simulink model "IEEE_39_bus_steady_state"  (R2021b)
settings: Solver=ode3  StartTime=0.0  StopTime=10  FixedStep=Ts  MaxStep=1/60  RelTol=1e-2  AbsTol=1e-1
PreLoadFcn:
  | Ts=50e-6; ssn_ieee39_params; dec=20;
InitFcn:
  | Ts=50e-6; ssn_ieee39_params; dec=20;
values from neighbouring files (symbols this model uses):
  f = 50    [ssn_ieee39_params_ctrl.m]
  fNom = f    (= 60)    [ssn_ieee39_params_ctrl.m]
  ILR = 5.02    [ssn_ieee39_params_ctrl.m]
  IQMIN = 0.1    [ssn_ieee39_params_ctrl.m]
  ISCLIM = 1    [ssn_ieee39_params_ctrl.m]
  ITFpu = 1.10    (= 1.1)    [ssn_ieee39_params_ctrl.m]
  K = 1    [ssn_ieee39_params_ctrl.m]
  K1 = 1    [ssn_ieee39_params_ctrl.m]
  K2 = 2    [ssn_ieee39_params_ctrl.m]
  KCL = 1.04    [ssn_ieee39_params_ctrl.m]
  KFB = 0    [ssn_ieee39_params_ctrl.m]
  KFF = 1    [ssn_ieee39_params_ctrl.m]
  KFIX = 1    [ssn_ieee39_params_ctrl.m]
  KG = 1    [ssn_ieee39_params_ctrl.m]
  KIA = 59.91    [ssn_ieee39_params_ctrl.m]
  KIOEX = 0.0303    [ssn_ieee39_params_ctrl.m]
  KIUEX = 0.0303    [ssn_ieee39_params_ctrl.m]
  KIUOEX = 1    [ssn_ieee39_params_ctrl.m]
  KIUUEX = 1    [ssn_ieee39_params_ctrl.m]
  KLR = 22.47    [ssn_ieee39_params_ctrl.m]
  KM = 1    [ssn_ieee39_params_ctrl.m]
  KOEL = 0.24    [ssn_ieee39_params_ctrl.m]
  Kp = 1    [ssn_ieee39_params_ctrl.m]
  KPA = 30    [ssn_ieee39_params_ctrl.m]
  KPOEL = 1    [ssn_ieee39_params_ctrl.m]
  KPOEX = 0    [ssn_ieee39_params_ctrl.m]
  KPUEX = 0    [ssn_ieee39_params_ctrl.m]
  KSCALE = 0.319    [ssn_ieee39_params_ctrl.m]
  KUF = 0    [ssn_ieee39_params_ctrl.m]
  KUI = 0.001    [ssn_ieee39_params_ctrl.m]
  KUL = 0.24    [ssn_ieee39_params_ctrl.m]
  s = 10    [ssn_ieee39_params_ctrl.m]
  TA = 0.01    [ssn_ieee39_params_ctrl.m]
  Tadj = 0    [ssn_ieee39_params_ctrl.m]
  taps = [1 1 1.07 1.07 1.009 1.025 1 1.025 1.025 1.025]*1    [ssn_ieee39_params_ctrl.m]
  TF = 0.02    [ssn_ieee39_params_ctrl.m]
  TG = 0.024    [ssn_ieee39_params_ctrl.m]
  TINV = 0    [ssn_ieee39_params_ctrl.m]
  TIT = 0.1    [ssn_ieee39_params_ctrl.m]
  TL_10_11_len = 14    [ssn_ieee39_params_ctrl.m]
  TL_10_13_len = 14    [ssn_ieee39_params_ctrl.m]
  TL_13_14_len = 32    [ssn_ieee39_params_ctrl.m]
  TL_14_15_len = 70    [ssn_ieee39_params_ctrl.m]
  TL_15_16_len = 31.5    [ssn_ieee39_params_ctrl.m]
  TL_16_17_len = 26    [ssn_ieee39_params_ctrl.m]
  TL_16_19_len = 61    [ssn_ieee39_params_ctrl.m]
  TL_16_21_len = 46    [ssn_ieee39_params_ctrl.m]
  TL_16_24_len = 15    [ssn_ieee39_params_ctrl.m]
  TL_17_18_len = 26    [ssn_ieee39_params_ctrl.m]
  TL_17_27_len = 59    [ssn_ieee39_params_ctrl.m]
  TL_1_2_len = 134    [ssn_ieee39_params_ctrl.m]
  TL_1_39_len = 105    [ssn_ieee39_params_ctrl.m]
  TL_21_22_len = 47    [ssn_ieee39_params_ctrl.m]
  TL_22_23_len = 33    [ssn_ieee39_params_ctrl.m]
  TL_24_23_len = 88    [ssn_ieee39_params_ctrl.m]
  TL_25_26_len = 101    [ssn_ieee39_params_ctrl.m]
  TL_26_27_len = 46.5    [ssn_ieee39_params_ctrl.m]
  TL_26_28_len = 151    [ssn_ieee39_params_ctrl.m]
  TL_26_29_len = 200    [ssn_ieee39_params_ctrl.m]
  TL_28_29_len = 48    [ssn_ieee39_params_ctrl.m]
  TL_2_25_len = 28    [ssn_ieee39_params_ctrl.m]
  TL_2_2_len = 49    [ssn_ieee39_params_ctrl.m]
  TL_3_18_len = 42    [ssn_ieee39_params_ctrl.m]
  TL_3_4_len = 53    [ssn_ieee39_params_ctrl.m]
  TL_4_14_len = 33    [ssn_ieee39_params_ctrl.m]
  TL_4_5_len = 32.5    [ssn_ieee39_params_ctrl.m]
  TL_5_6_len = 14    [ssn_ieee39_params_ctrl.m]
  TL_5_8_len = 32    [ssn_ieee39_params_ctrl.m]
  TL_6_11_len = 26.5    [ssn_ieee39_params_ctrl.m]
  TL_6_7_len = 25.5    [ssn_ieee39_params_ctrl.m]
  TL_7_8_len = 15    [ssn_ieee39_params_ctrl.m]
  TL_8_9_len = 93    [ssn_ieee39_params_ctrl.m]
  TL_9_39_len = 136    [ssn_ieee39_params_ctrl.m]
  TOEL = 5.00    (= 5)    [ssn_ieee39_params_ctrl.m]
  TQREF = 0    [ssn_ieee39_params_ctrl.m]
  TQSCL = 0.012    [ssn_ieee39_params_ctrl.m]
  Ts_PMU = 1/1000    (= 0.001)    [ssn_ieee39_params_ctrl.m]
  TU1 = 0    [ssn_ieee39_params_ctrl.m]
  TU2 = 0    [ssn_ieee39_params_ctrl.m]
  TU3 = 0    [ssn_ieee39_params_ctrl.m]
  TU4 = 0    [ssn_ieee39_params_ctrl.m]
  TUL = 0    [ssn_ieee39_params_ctrl.m]
  TUP = 0.050    (= 0.05)    [ssn_ieee39_params_ctrl.m]
  TUQ = .005    (= 0.005)    [ssn_ieee39_params_ctrl.m]
  TUV = 0.2    [ssn_ieee39_params_ctrl.m]
  VAAMAX = VAMAX    (= 7.05)    [ssn_ieee39_params_ctrl.m]
  VAMAX = 7.05    [ssn_ieee39_params_ctrl.m]
  VAMIN = -6.11    [ssn_ieee39_params_ctrl.m]
  VBMAX = 999    [ssn_ieee39_params_ctrl.m]
  VF = 0    [ssn_ieee39_params_ctrl.m]
  VFB = 0    [ssn_ieee39_params_ctrl.m]
  VMMAX = 7.05    [ssn_ieee39_params_ctrl.m]
  VMMIN = -6.11    [ssn_ieee39_params_ctrl.m]
  VOELmax1 = 0.2353    [ssn_ieee39_params_ctrl.m]
  VOELmax2 = 0.0    (= 0)    [ssn_ieee39_params_ctrl.m]
  VOELmin1 = -0.24    [ssn_ieee39_params_ctrl.m]
  VOELmin2 = -1.0    (= -1)    [ssn_ieee39_params_ctrl.m]
  VRMAX = 7.05    [ssn_ieee39_params_ctrl.m]
  VRMIN = -6.11    [ssn_ieee39_params_ctrl.m]
  VSCLmax = 0.20    (= 0.2)    [ssn_ieee39_params_ctrl.m]
  VSCLmin = -0.10    (= -0.1)    [ssn_ieee39_params_ctrl.m]
  VUELmax1 = 1    [ssn_ieee39_params_ctrl.m]
  VUELmax2 = 1    [ssn_ieee39_params_ctrl.m]
  VUELmin1 = -1    [ssn_ieee39_params_ctrl.m]
  VUELmin2 = -1    [ssn_ieee39_params_ctrl.m]
  VUImax = 1    [ssn_ieee39_params_ctrl.m]
  VUImin = -1    [ssn_ieee39_params_ctrl.m]
undefined symbols (not defined in the file or in its folder): D1, Delta, MOV_segment9, powergui
libraries: spsThreePhaseVIMeasurementLib x43, slpidlib x40, op_dpl_lib x32, powerlib_extras x30, simulink_extras x20, spsST2AModel x20, spsThreePhaseParallelRLCLoadLib x20, spsThreePhaseTransformerTwoWindingsLib x13, spsSynchronousMachinepuStandardLib x10, simulink x10, spsPower3phInstantaneousLib x10, spsThreePhasePISectionLineLib x4
(part 5 of 15)

== system IEEE_39_bus_steady_state/SM_master/G7/G7 ==
  note: Rotor Speed
  note: Rotor Speed Reference
  note: SM Measurement Signal
  note: Active Power
  note: Field Current
  note: Voltage Reference
  note: Stator Voltage
  note: Reactive Power
  note: Stator Current
  note: Field Voltage (Vf)
  note: Mechanical
      | Power (Pm)
  note: Measurement Outputs
  note: Rotor Speed
  note: Active Power
  note: Stator Voltage
  note: Stator Current
  note: Field Current
  note: Reactive Power
  wref (pu) : Inport
  Vref (pu) : Inport  Port=2
  Generator Measurements (Output) : Subsystem
  Governor model with Droop : Subsystem
  Ground7 : Ground
  ST6C EXCITER-1 : Subsystem
  Synchronous Machine : spsSynchronousMachinepuStandardLib/Synchronous Machine pu Standard  PresetModel=No  MechanicalLoad=Mechanical power Pm  ShowDetailedParameters=on  RotorType=Salient-pole  Units=per unit standard parameters  MeasurementBus=off  NominalParameters="[ Pn  Vn   f ]"  Reactances1=[ 31 32 33 34 35 36 37 ]  Reactances2=[ 1.305, 0.296, 0.252, 0.474, 0.243, 0.18 ]  dAxisTimeConstants=Short-circuit  qAxisTimeConstants=Open-circuit  TimeConstants1=[]  TimeConstants2=[]  TimeConstants3=[]  TimeConstants4=[]  TimeConstants5=[ 1.01, 0.053, 0.1 ]  TimeConstants6=[]  TimeConstants7=[]  TimeConstants8=[]  StatorResistance=2.8544e-3  Mechanical=[H1 0 2]  PolePairs=2  InitialConditions=[0 -62.5202 1.01055 1.01055 1.01055 8.25986 -111.74 128.26 1.32748]  SetSaturation=off  Saturation=[0.6404,0.7127,0.8441,0.9214,0.9956,1.082,1.19,1.316,1.457;0.7,0.7698,0.8872,0.9466,0.9969,1.046,1.1,1.151,1.201]  LoadFlowParameters=[1 150000000 0 0]  TsPowergui=0  TsBlock=-1  IterativeModel=Trapezoidal non iterative  IterativeDiscreteModel=Trapezoidal non iterative  BusType=PV  Pref=42e6  Qref=0  Qmin=-50000000  Qmax=50000000  PLF=0  QLF=0
      settings: SourceProductBaseCode=PS
  A : PMIOPort  Side=Right
  B : PMIOPort  Port=2  Side=Right
  C : PMIOPort  Port=3  Side=Right
  sm1 : Outport  VectorParamsAs1DForOutWhenUnconnected=off
  wires:
  [PT1st] -> Governor model with Droop/3(Input)
  [Ifd1st] -> ST6C EXCITER-1/4(Ifd)
  [Vt1st] -> ST6C EXCITER-1/2(Vt)
  [wm1] -> Governor model with Droop/2(w (pu))
  Generator Measurements (Output)/3(Vt) -> [Vt1st]
  Generator Measurements (Output)/6(PT) -> [PT1st]
  Generator Measurements (Output)/7(QT) -> [QT1st]
  Generator Measurements (Output)/1(sm) -> sm1/1
  Generator Measurements (Output)/5(It) -> [It1st]
  Generator Measurements (Output)/4(Ifd) -> [Ifd1st]
  Generator Measurements (Output)/2(wm) -> [wm1]
  ST6C EXCITER-1/1(Efd) -> Synchronous Machine/2, [Efd1st]
  [PT1st] -> ST6C EXCITER-1/7(PT)
  [It1st] -> ST6C EXCITER-1/3(It)
  [QT1st] -> ST6C EXCITER-1/6(QT)
  Ground7/1 -> ST6C EXCITER-1/5(Vstab)
  wref (pu)/1 -> Governor model with Droop/1(wref (pu)1)
  Governor model with Droop/1(Pmec (pu)) -> Synchronous Machine/1
  Vref (pu)/1 -> ST6C EXCITER-1/1(Vref)
  Synchronous Machine/1 -> Generator Measurements (Output)/1(m)
  connections:
  A/RConn1 -- Synchronous Machine/RConn1
  C/RConn1 -- Synchronous Machine/RConn3
  B/RConn1 -- Synchronous Machine/RConn2

== system IEEE_39_bus_steady_state/SM_master/G8/ G8 ==
  note: Reactive Power
  note: Field Current
  note: Stator Current
  note: Stator Voltage
  note: Active Power
  note: Rotor Speed
  note: Measurement Outputs
  note: Mechanical
      | Power (PU)
  note: Field Voltage (Vf PU)
  note: Stator Current
  note: Reactive Power
  note: Stator Voltage
  note: Voltage Reference
  note: Field Current
  note: Active Power
  note: SM Measurement Signal
  note: Rotor Speed Reference
  note: Rotor Speed
  wref (pu) : Inport
  Vref (pu) : Inport  Port=2
  "Generator Measurements " : Subsystem
  "Governor model " : Subsystem
  Ground7 : Ground
  ST6C EXCITER-1 : Subsystem
  Synchronous Machine : spsSynchronousMachinepuStandardLib/Synchronous Machine pu Standard  PresetModel=No  MechanicalLoad=Mechanical power Pm  ShowDetailedParameters=on  RotorType=Salient-pole  Units=per unit standard parameters  MeasurementBus=off  NominalParameters="[ Pn  Vn   f ]"  Reactances1=[ 31 32 33 34 35 36 37 ]  Reactances2=[ 1.305, 0.296, 0.252, 0.474, 0.243, 0.18 ]  dAxisTimeConstants=Short-circuit  qAxisTimeConstants=Open-circuit  TimeConstants1=[]  TimeConstants2=[]  TimeConstants3=[]  TimeConstants4=[]  TimeConstants5=[ 1.01, 0.053, 0.1 ]  TimeConstants6=[]  TimeConstants7=[]  TimeConstants8=[]  StatorResistance=2.8544e-3  Mechanical=[H1 0 2]  PolePairs=2  InitialConditions=[0 -62.5202 1.01055 1.01055 1.01055 8.25986 -111.74 128.26 1.32748]  SetSaturation=off  Saturation=[0.6404,0.7127,0.8441,0.9214,0.9956,1.082,1.19,1.316,1.457;0.7,0.7698,0.8872,0.9466,0.9969,1.046,1.1,1.151,1.201]  LoadFlowParameters=[1 150000000 0 0]  TsPowergui=0  TsBlock=-1  IterativeModel=Trapezoidal non iterative  IterativeDiscreteModel=Trapezoidal non iterative  BusType=PV  Pref=42e6  Qref=0  Qmin=-50000000  Qmax=50000000  PLF=0  QLF=0
      settings: SourceProductBaseCode=PS
  A : PMIOPort  Side=Right
  B : PMIOPort  Port=2  Side=Right
  C : PMIOPort  Port=3  Side=Right
  sm1 : Outport  VectorParamsAs1DForOutWhenUnconnected=off
  wires:
  Synchronous Machine/1 -> "Generator Measurements "/1(m)
  Vref (pu)/1 -> ST6C EXCITER-1/1(Vref)
  "Governor model "/1(Pmec (pu)) -> Synchronous Machine/1
  wref (pu)/1 -> "Governor model "/1(wref (pu)1)
  Ground7/1 -> ST6C EXCITER-1/5(Vstab)
  [QT1st] -> ST6C EXCITER-1/6(QT)
  [It1st] -> ST6C EXCITER-1/3(It)
  [PT1st] -> ST6C EXCITER-1/7(PT)
  ST6C EXCITER-1/1(Efd) -> [Efd1st], Synchronous Machine/2
  "Generator Measurements "/2(wm) -> [wm1]
  "Generator Measurements "/4(Ifd) -> [Ifd1st]
  "Generator Measurements "/5(It) -> [It1st]
  "Generator Measurements "/1(sm) -> sm1/1
  "Generator Measurements "/7(QT) -> [QT1st]
  "Generator Measurements "/6(PT) -> [PT1st]
  "Generator Measurements "/3(Vt) -> [Vt1st]
  [wm1] -> "Governor model "/2(w (pu))
  [Vt1st] -> ST6C EXCITER-1/2(Vt)
  [Ifd1st] -> ST6C EXCITER-1/4(Ifd)
  [PT1st] -> "Governor model "/3(Input)
  connections:
  B/RConn1 -- Synchronous Machine/RConn2
  C/RConn1 -- Synchronous Machine/RConn3
  A/RConn1 -- Synchronous Machine/RConn1

== system IEEE_39_bus_steady_state/SM_master/G9/G9 ==
  note: Rotor Speed
  note: Rotor Speed Reference
  note: SM Measurement Signal
  note: Active Power
  note: Field Current
  note: Voltage Reference
  note: Stator Voltage
  note: Reactive Power
  note: Stator Current
  note: Field Voltage (Vf)
  note: Mechanical
      | Power (Pm)
  note: Measurement Outputs
  note: Rotor Speed
  note: Active Power
  note: Stator Voltage
  note: Stator Current
  note: Field Current
  note: Reactive Power
  wref (pu) : Inport
  Vref (pu) : Inport  Port=2
  Generator Measurements (Output) : Subsystem
  Governor model with Droop : Subsystem
  Ground7 : Ground
  ST6C EXCITER-1 : Subsystem
  Synchronous Machine : spsSynchronousMachinepuStandardLib/Synchronous Machine pu Standard  PresetModel=No  MechanicalLoad=Mechanical power Pm  ShowDetailedParameters=on  RotorType=Salient-pole  Units=per unit standard parameters  MeasurementBus=off  NominalParameters="[ Pn  Vn   f ]"  Reactances1=[ 31 32 33 34 35 36 37 ]  Reactances2=[ 1.305, 0.296, 0.252, 0.474, 0.243, 0.18 ]  dAxisTimeConstants=Short-circuit  qAxisTimeConstants=Open-circuit  TimeConstants1=[]  TimeConstants2=[]  TimeConstants3=[]  TimeConstants4=[]  TimeConstants5=[ 1.01, 0.053, 0.1 ]  TimeConstants6=[]  TimeConstants7=[]  TimeConstants8=[]  StatorResistance=2.8544e-3  Mechanical=[H1 0 2]  PolePairs=2  InitialConditions=[0 -62.5202 1.01055 1.01055 1.01055 8.25986 -111.74 128.26 1.32748]  SetSaturation=off  Saturation=[0.6404,0.7127,0.8441,0.9214,0.9956,1.082,1.19,1.316,1.457;0.7,0.7698,0.8872,0.9466,0.9969,1.046,1.1,1.151,1.201]  LoadFlowParameters=[1 150000000 0 0]  TsPowergui=0  TsBlock=-1  IterativeModel=Trapezoidal non iterative  IterativeDiscreteModel=Trapezoidal non iterative  BusType=PV  Pref=42e6  Qref=0  Qmin=-50000000  Qmax=50000000  PLF=0  QLF=0
      settings: SourceProductBaseCode=PS
  A : PMIOPort  Side=Right
  B : PMIOPort  Port=2  Side=Right
  C : PMIOPort  Port=3  Side=Right
  sm1 : Outport  VectorParamsAs1DForOutWhenUnconnected=off
  wires:
  [PT1st] -> Governor model with Droop/3(Input)
  [Ifd1st] -> ST6C EXCITER-1/4(Ifd)
  [Vt1st] -> ST6C EXCITER-1/2(Vt)
  [wm1] -> Governor model with Droop/2(w (pu))
  Generator Measurements (Output)/3(Vt) -> [Vt1st]
  Generator Measurements (Output)/6(PT) -> [PT1st]
  Generator Measurements (Output)/7(QT) -> [QT1st]
  Generator Measurements (Output)/1(sm) -> sm1/1
  Generator Measurements (Output)/5(It) -> [It1st]
  Generator Measurements (Output)/4(Ifd) -> [Ifd1st]
  Generator Measurements (Output)/2(wm) -> [wm1]
  ST6C EXCITER-1/1(Efd) -> Synchronous Machine/2, [Efd1st]
  [PT1st] -> ST6C EXCITER-1/7(PT)
  [It1st] -> ST6C EXCITER-1/3(It)
  [QT1st] -> ST6C EXCITER-1/6(QT)
  Ground7/1 -> ST6C EXCITER-1/5(Vstab)
  wref (pu)/1 -> Governor model with Droop/1(wref (pu)1)
  Governor model with Droop/1(Pmec (pu)) -> Synchronous Machine/1
  Vref (pu)/1 -> ST6C EXCITER-1/1(Vref)
  Synchronous Machine/1 -> Generator Measurements (Output)/1(m)
  connections:
  A/RConn1 -- Synchronous Machine/RConn1
  C/RConn1 -- Synchronous Machine/RConn3
  B/RConn1 -- Synchronous Machine/RConn2

== system IEEE_39_bus_steady_state/powergui/EquivalentModel1/Sources ==
  Mux : Mux  Inputs=[1 1 1 1 1 1 1 1 1]
  u : Outport  VectorParamsAs1DForOutWhenUnconnected=off
  wires:
  Mux/1 -> u/1
  [T80_6490_9326860332146] -> Mux/1
  [T80_6491_9328226718070] -> Mux/2
  [T80_6492_9329829299994] -> Mux/3
  [T80_6492_9324012370568] -> Mux/4
  [T80_6493_9325375056125] -> Mux/5
  [T80_6494_9326973937682] -> Mux/6
  [T80_6492_9323337455089] -> Mux/7
  [T80_6493_9324700180633] -> Mux/8
  [T80_6494_9326299102177] -> Mux/9

== system IEEE_39_bus_steady_state/powergui/EquivalentModel1/Yout ==
  v,i : Inport
  Demux : Demux  Outputs=[1 1 1 1 1 1 1 1 1 1 1 1]
  tag scope: T60_4973_5506940896565=global, T60_4974_5509192109658=global, T60_4975_5512020233025=global, T83_6848_11089873256421=global, T83_6849_11090645481369=global, T83_6850_11085613834681=global, T83_6850_11086254604711=global, T83_6850_11091651495475=global, T83_6851_11086382615169=global, T83_6851_11087023347570=global, T83_6852_11087385184813=global, T83_6852_11088025879586=global
  wires:
  v,i/1 -> Demux/1
  Demux/1 -> [T60_4973_5506940896565]
  Demux/2 -> [T60_4975_5512020233025]
  Demux/3 -> [T60_4974_5509192109658]
  Demux/4 -> [T83_6848_11089873256421]
  Demux/5 -> [T83_6849_11090645481369]
  Demux/6 -> [T83_6850_11091651495475]
  Demux/7 -> [T83_6850_11086254604711]
  Demux/8 -> [T83_6851_11087023347570]
  Demux/9 -> [T83_6852_11088025879586]
  Demux/10 -> [T83_6850_11085613834681]
  Demux/11 -> [T83_6851_11086382615169]
  Demux/12 -> [T83_6852_11087385184813]

== system IEEE_39_bus_steady_state/powergui/EquivalentModel10/Sources ==
  Mux : Mux  Inputs=[1 1 1 1 1 1]
  u : Outport  VectorParamsAs1DForOutWhenUnconnected=off
  wires:
  Mux/1 -> u/1
  [T80_6485_9333533310861] -> Mux/1
  [T80_6486_9334909607494] -> Mux/2
  [T80_6487_9336522100127] -> Mux/3
  [T80_6488_9329887439771] -> Mux/4
  [T80_6489_9331257526062] -> Mux/5
  [T80_6490_9332863808353] -> Mux/6

== system IEEE_39_bus_steady_state/powergui/EquivalentModel10/Yout ==
  v,i : Inport
  Demux : Demux  Outputs=[1 1 1 1 1 1 1 1 1]
  tag scope: T60_4971_5508420908090=global, T60_4972_5510675995873=global, T60_4973_5513508227489=global, T83_6843_11098646092448=global, T83_6844_11099427643491=global, T83_6845_11100442983691=global, T83_6846_11093664659533=global, T83_6847_11094440366571=global, T83_6848_11095449862765=global
  wires:
  v,i/1 -> Demux/1
  Demux/1 -> [T60_4971_5508420908090]
  Demux/2 -> [T60_4973_5513508227489]
  Demux/3 -> [T60_4972_5510675995873]
  Demux/4 -> [T83_6843_11098646092448]
  Demux/5 -> [T83_6844_11099427643491]
  Demux/6 -> [T83_6845_11100442983691]
  Demux/7 -> [T83_6846_11093664659533]
  Demux/8 -> [T83_6847_11094440366571]
  Demux/9 -> [T83_6848_11095449862765]

== system IEEE_39_bus_steady_state/powergui/EquivalentModel11/Sources ==
  Mux : Mux  Inputs=[1 1 1 1 1 1 1 1 1 1 1 1 1 1 1]
  u : Outport  VectorParamsAs1DForOutWhenUnconnected=off
  wires:
  Mux/1 -> u/1
  [T80_6487_9330330163669] -> Mux/1
  [T80_6488_9331702759935] -> Mux/2
  [T80_6489_9333311552201] -> Mux/3
  [T80_6489_9327306162525] -> Mux/4
  [T80_6490_9328675058424] -> Mux/5
  [T80_6491_9330280150323] -> Mux/6
  [T80_6491_9325043360348] -> Mux/7
  [T80_6492_9326408355943] -> Mux/8
  [T80_6493_9328009547538] -> Mux/9
  [T80_6484_9334657162593] -> Mux/10
  [T80_6485_9336035849239] -> Mux/11
  [T80_6486_9337650731884] -> Mux/12
  [T80_6487_9329601153036] -> Mux/13
  [T80_6488_9330973989226] -> Mux/14
  [T80_6489_9332583021416] -> Mux/15

== system IEEE_39_bus_steady_state/powergui/EquivalentModel11/Yout ==
  v,i : Inport
  Demux : Demux  Outputs=[1 1 1 1 1 1 1 1 1 1 1 1 1 1 1 1 1 1]
  tag scope: T60_4972_5507634085661=global, T60_4973_5509887236099=global, T60_4974_5512717413590=global, T83_6842_11100294262903=global, T83_6843_11101078062977=global, T83_6844_11102095652207=global, T83_6845_11094039231572=global, T83_6845_11094684822589=global, T83_6846_11094817526297=global, T83_6846_11095462891543=global, T83_6847_11090896304132=global, T83_6847_11095829610179=global, T83_6847_11096474749653=global, T83_6848_11091670890996=global, T83_6849_11087794022709=global, T83_6849_11092679267017=global, T83_6850_11088564939342=global, T83_6851_11089569645131=global
  wires:
  v,i/1 -> Demux/1
  Demux/1 -> [T60_4972_5507634085661]
  Demux/2 -> [T60_4974_5512717413590]
  Demux/3 -> [T60_4973_5509887236099]
  Demux/4 -> [T83_6845_11094684822589]
  Demux/5 -> [T83_6846_11095462891543]
  Demux/6 -> [T83_6847_11096474749653]
  Demux/7 -> [T83_6847_11090896304132]
  Demux/8 -> [T83_6848_11091670890996]
  Demux/9 -> [T83_6849_11092679267017]
  Demux/10 -> [T83_6849_11087794022709]
  Demux/11 -> [T83_6850_11088564939342]
  Demux/12 -> [T83_6851_11089569645131]
  Demux/13 -> [T83_6842_11100294262903]
  Demux/14 -> [T83_6843_11101078062977]
  Demux/15 -> [T83_6844_11102095652207]
  Demux/16 -> [T83_6845_11094039231572]
  Demux/17 -> [T83_6846_11094817526297]
  Demux/18 -> [T83_6847_11095829610179]

== system IEEE_39_bus_steady_state/powergui/EquivalentModel12/Sources ==
  Mux : Mux  Inputs=[1 1 1 1 1 1]
  u : Outport  VectorParamsAs1DForOutWhenUnconnected=off
  wires:
  Mux/1 -> u/1
  [T80_6491_9324461307429] -> Mux/1
  [T80_6492_9325826502960] -> Mux/2
  [T80_6493_9327427894492] -> Mux/3
  [T79_6439_9116019234382] -> Mux/4
  [T79_6440_9117301486793] -> Mux/5
  [T79_6441_9118816569838] -> Mux/6

== system IEEE_39_bus_steady_state/powergui/EquivalentModel12/Yout ==
  v,i : Inport
  Demux : Demux  Outputs=[1 1 1 1 1 1 1 1 1]
  tag scope: T60_4974_5506341340802=global, T60_4975_5508590616551=global, T60_4976_5511416685794=global, T82_6797_10841513870003=global, T82_6798_10842206375369=global, T82_6799_10843129315857=global, T83_6849_11087280537076=global, T83_6850_11088051641851=global, T83_6851_11089056535783=global
  wires:
  v,i/1 -> Demux/1
  Demux/1 -> [T60_4974_5506341340802]
  Demux/2 -> [T60_4976_5511416685794]
  Demux/3 -> [T60_4975_5508590616551]
  Demux/4 -> [T83_6849_11087280537076]
  Demux/5 -> [T83_6850_11088051641851]
  Demux/6 -> [T83_6851_11089056535783]
  Demux/7 -> [T82_6797_10841513870003]
  Demux/8 -> [T82_6798_10842206375369]
  Demux/9 -> [T82_6799_10843129315857]

== system IEEE_39_bus_steady_state/powergui/EquivalentModel13/Sources ==
  Mux : Mux  Inputs=[2 2 1 1 1]
  u : Outport  VectorParamsAs1DForOutWhenUnconnected=off
  wires:
  Mux/1 -> u/1
  [T69_5984_8388252215439] -> Mux/1
  [T69_5986_8384514256884] -> Mux/2
  [T80_6492_9324594255639] -> Mux/3
  [T80_6493_9325956741259] -> Mux/4
  [T80_6494_9327555422880] -> Mux/5

== system IEEE_39_bus_steady_state/powergui/EquivalentModel13/Yout ==
  v,i : Inport
  Demux : Demux  Outputs=[2 2 1 1 1 1 1 1 1 1 1 1 1 1 1 1 1 1 1 1 1 1 1]
  tag scope: T59_4890_5390840927732=global, T59_4891_5393348121537=global, T59_4892_5396002976359=global, T59_4894_5386756332279=global, T59_4895_5389255398556=global, T59_4896_5391902125850=global, T60_4967_5512515441523=global, T60_4968_5511258904347=global, T60_4968_5514778326203=global, T60_4969_5513519851684=global, T60_4969_5517618824701=global, T60_4970_5516358296056=global, T60_4972_5506889918124=global, T60_4973_5509143163602=global, T60_4974_5511973441862=global, T60_4975_5505835418373=global, T60_4976_5508082756777=global, T60_4977_5510906771895=global, T69_5979_8319434027570=global, T69_5981_8315716887242=global, T83_6850_11086767934481=global, T83_6851_11087536489198=global, T83_6852_11088538833071=global
  wires:
  v,i/1 -> Demux/1
  Demux/1 -> [T69_5979_8319434027570]
  Demux/2 -> [T69_5981_8315716887242]
  Demux/3 -> [T60_4975_5505835418373]
  Demux/4 -> [T60_4977_5510906771895]
  Demux/5 -> [T60_4976_5508082756777]
  Demux/6 -> [T60_4967_5512515441523]
  Demux/7 -> [T60_4969_5517618824701]
  Demux/8 -> [T60_4968_5514778326203]
  Demux/9 -> [T60_4968_5511258904347]
  Demux/10 -> [T60_4970_5516358296056]
  Demux/11 -> [T60_4969_5513519851684]
  Demux/12 -> [T60_4972_5506889918124]
  Demux/13 -> [T60_4974_5511973441862]
  Demux/14 -> [T60_4973_5509143163602]
  Demux/15 -> [T83_6850_11086767934481]
  Demux/16 -> [T83_6851_11087536489198]
  Demux/17 -> [T83_6852_11088538833071]
  Demux/18 -> [T59_4890_5390840927732]
  Demux/19 -> [T59_4891_5393348121537]
  Demux/20 -> [T59_4892_5396002976359]
  Demux/21 -> [T59_4894_5386756332279]
  Demux/22 -> [T59_4895_5389255398556]
  Demux/23 -> [T59_4896_5391902125850]

== system IEEE_39_bus_steady_state/powergui/EquivalentModel14/Sources ==
  Mux : Mux  Inputs=[1 1 1 1 1 1]
  u : Outport  VectorParamsAs1DForOutWhenUnconnected=off
  wires:
  Mux/1 -> u/1
  [T80_6485_9334219551606] -> Mux/1
  [T80_6486_9335595728277] -> Mux/2
  [T80_6487_9337208100948] -> Mux/3
  [T80_6481_9340267199468] -> Mux/4
  [T80_6482_9341650976810] -> Mux/5
  [T80_6483_9343270950152] -> Mux/6

== system IEEE_39_bus_steady_state/powergui/EquivalentModel14/Yout ==
  v,i : Inport
  Demux : Demux  Outputs=[1 1 1 1 1 1 1 1 1]
  tag scope: T60_4970_5509026729997=global, T60_4971_5511283802644=global, T60_4972_5514118138768=global, T83_6839_11106903646101=global, T83_6840_11107692236579=global, T83_6841_11108714616215=global, T83_6843_11099278847658=global, T83_6844_11100060285815=global, T83_6845_11101075513130=global
  wires:
  v,i/1 -> Demux/1
  Demux/1 -> [T60_4970_5509026729997]
  Demux/2 -> [T60_4972_5514118138768]
  Demux/3 -> [T60_4971_5511283802644]
  Demux/4 -> [T83_6843_11099278847658]
  Demux/5 -> [T83_6844_11100060285815]
  Demux/6 -> [T83_6845_11101075513130]
  Demux/7 -> [T83_6839_11106903646101]
  Demux/8 -> [T83_6840_11107692236579]
  Demux/9 -> [T83_6841_11108714616215]

== system IEEE_39_bus_steady_state/powergui/EquivalentModel15/Sources ==
  Mux : Mux  Inputs=[2 1 1 1 1 1 1]
  u : Outport  VectorParamsAs1DForOutWhenUnconnected=off
  wires:
  Mux/1 -> u/1
  [T69_5990_8377556419160] -> Mux/1
  [T80_6484_9336085689543] -> Mux/2
  [T80_6485_9337463256543] -> Mux/3
  [T80_6486_9339077019543] -> Mux/4
  [T80_6486_9332196927467] -> Mux/5
  [T80_6487_9333570994036] -> Mux/6
  [T80_6488_9335181256606] -> Mux/7

== system IEEE_39_bus_steady_state/powergui/EquivalentModel15/Yout ==
  v,i : Inport
  Demux : Demux  Outputs=[2 1 1 1 1 1 1 1 1 1 1 1 1 1 1 1]
  tag scope: T59_4895_5385947963022=global, T59_4896_5388444984880=global, T59_4897_5391089667756=global, T60_4973_5506006366203=global, T60_4974_5505216447616=global, T60_4974_5508257674336=global, T60_4975_5507465818404=global, T60_4975_5511085898472=global, T60_4976_5510291988415=global, T69_5985_8308800685972=global, T83_6842_11101405629803=global, T83_6843_11102188376277=global, T83_6844_11096831067105=global, T83_6844_11103204911907=global, T83_6845_11097610519633=global, T83_6846_11098623761316=global
  wires:
  v,i/1 -> Demux/1
  Demux/1 -> [T69_5985_8308800685972]
  Demux/2 -> [T60_4973_5506006366203]
  Demux/3 -> [T60_4975_5511085898472]
  Demux/4 -> [T60_4974_5508257674336]
  Demux/5 -> [T60_4974_5505216447616]
  Demux/6 -> [T60_4976_5510291988415]
  Demux/7 -> [T60_4975_5507465818404]
  Demux/8 -> [T83_6842_11101405629803]
  Demux/9 -> [T83_6843_11102188376277]
  Demux/10 -> [T83_6844_11103204911907]
  Demux/11 -> [T83_6844_11096831067105]
  Demux/12 -> [T83_6845_11097610519633]
  Demux/13 -> [T83_6846_11098623761316]
  Demux/14 -> [T59_4895_5385947963022]
  Demux/15 -> [T59_4896_5388444984880]
  Demux/16 -> [T59_4897_5391089667756]

== system IEEE_39_bus_steady_state/powergui/EquivalentModel16/Sources ==
  Mux : Mux  Inputs=[1 1 1 1 1 1]
  u : Outport  VectorParamsAs1DForOutWhenUnconnected=off
  wires:
  Mux/1 -> u/1
  [T80_6488_9329158630555] -> Mux/1
  [T80_6489_9330528956771] -> Mux/2
  [T80_6490_9332135478986] -> Mux/3
  [T80_6485_9332636309897] -> Mux/4
  [T80_6486_9334012886441] -> Mux/5
  [T80_6487_9335625658986] -> Mux/6

== system IEEE_39_bus_steady_state/powergui/EquivalentModel16/Yout ==
  v,i : Inport
  Demux : Demux  Outputs=[1 1 1 1 1 1 1 1 1]
  tag scope: T60_4971_5507867103379=global, T60_4972_5510122286201=global, T60_4973_5512954618585=global, T83_6843_11097848127299=global, T83_6844_11098629941743=global, T83_6845_11099645545342=global, T83_6846_11093019255551=global, T83_6847_11093795188360=global, T83_6848_11094804910326=global
  wires:
  v,i/1 -> Demux/1
  Demux/1 -> [T60_4971_5507867103379]
  Demux/2 -> [T60_4973_5512954618585]
  Demux/3 -> [T60_4972_5510122286201]
  Demux/4 -> [T83_6846_11093019255551]
  Demux/5 -> [T83_6847_11093795188360]
  Demux/6 -> [T83_6848_11094804910326]
  Demux/7 -> [T83_6843_11097848127299]
  Demux/8 -> [T83_6844_11098629941743]
  Demux/9 -> [T83_6845_11099645545342]

== system IEEE_39_bus_steady_state/powergui/EquivalentModel17/Sources ==
  Mux : Mux  Inputs=[2 1 1 1 1 1 1]
  u : Outport  VectorParamsAs1DForOutWhenUnconnected=off
  wires:
  Mux/1 -> u/1
  [T70_6024_8653727448673] -> Mux/1
  [T80_6489_9326361811241] -> Mux/2
  [T80_6490_9327730787114] -> Mux/3
  [T80_6491_9329335958987] -> Mux/4
  [T79_6435_9120663979799] -> Mux/5
  [T79_6436_9121954368614] -> Mux/6
  [T79_6437_9123477588062] -> Mux/7

== system IEEE_39_bus_steady_state/powergui/EquivalentModel17/Yout ==
  v,i : Inport
  Demux : Demux  Outputs=[2 1 1 1 1 1 1 1 1 1 1 1 1 1 1 1]
  tag scope: T59_4897_5384616885523=global, T59_4898_5387109818545=global, T59_4899_5389750412583=global, T60_4972_5507169088980=global, T60_4973_5509422286938=global, T60_4974_5512252514814=global, T60_4975_5504520162362=global, T60_4976_5506767595805=global, T60_4977_5509591711692=global, T70_6019_8583423964389=global, T82_6793_10847905710015=global, T82_6794_10848605866113=global, T82_6795_10849536457332=global, T83_6847_11090005414928=global, T83_6848_11090780077050=global, T83_6849_11091788528328=global
  wires:
  v,i/1 -> Demux/1
  Demux/1 -> [T70_6019_8583423964389]
  Demux/2 -> [T60_4972_5507169088980]
  Demux/3 -> [T60_4974_5512252514814]
  Demux/4 -> [T60_4973_5509422286938]
  Demux/5 -> [T60_4975_5504520162362]
  Demux/6 -> [T60_4977_5509591711692]
  Demux/7 -> [T60_4976_5506767595805]
  Demux/8 -> [T83_6847_11090005414928]
  Demux/9 -> [T83_6848_11090780077050]
  Demux/10 -> [T83_6849_11091788528328]
  Demux/11 -> [T82_6793_10847905710015]
  Demux/12 -> [T82_6794_10848605866113]
  Demux/13 -> [T82_6795_10849536457332]
  Demux/14 -> [T59_4897_5384616885523]
  Demux/15 -> [T59_4898_5387109818545]
  Demux/16 -> [T59_4899_5389750412583]

== system IEEE_39_bus_steady_state/powergui/EquivalentModel18/Sources ==
  Mux : Mux  Inputs=[1 1 1 1 1 1 1 1 1 1 1 1]
  u : Outport  VectorParamsAs1DForOutWhenUnconnected=off
  wires:
  Mux/1 -> u/1
  [T80_6490_9325916048000] -> Mux/1
  [T80_6491_9327282513899] -> Mux/2
  [T80_6492_9328885175797] -> Mux/3
  [T81_6536_9547731076278] -> Mux/4
  [T81_6537_9549191642790] -> Mux/5
  [T81_6538_9550891771031] -> Mux/6
  [T80_6492_9322149322264] -> Mux/7
  [T80_6493_9323512647619] -> Mux/8
  [T80_6494_9325112168973] -> Mux/9
  [T80_6493_9321065804226] -> Mux/10
  [T80_6494_9322427179429] -> Mux/11
  [T80_6495_9324024750631] -> Mux/12

== system IEEE_39_bus_steady_state/powergui/EquivalentModel18/Yout ==
  v,i : Inport
  Demux : Demux  Outputs=[1 1 1 1 1 1 1 1 1 1 1 1 1 1 1 1 1 1 1 1 1]
  tag scope: T60_4973_5506380718472=global, T60_4974_5508631979085=global, T60_4975_5511460152836=global, T83_6848_11088982429562=global, T83_6849_11089754729768=global, T83_6850_11084610973670=global, T83_6850_11090760819130=global, T83_6851_11083106068569=global, T83_6851_11085380318587=global, T83_6852_11083873578369=global, T83_6852_11086383452659=global, T83_6853_11084874877326=global, T84_6894_11350402720670=global, T84_6895_11351264229999=global, T84_6896_11352362883137=global, T85_7290_11482635956345=global, T85_7291_11486699929756=global, T85_7292_11490998257050=global, T85_7302_11561671089655=global, T85_7303_11565702456143=global, T85_7304_11569968176513=global
  wires:
  v,i/1 -> Demux/1
  Demux/1 -> [T60_4973_5506380718472]
  Demux/2 -> [T60_4975_5511460152836]
  Demux/3 -> [T60_4974_5508631979085]
  Demux/4 -> [T83_6848_11088982429562]
  Demux/5 -> [T83_6849_11089754729768]
  Demux/6 -> [T83_6850_11090760819130]
  Demux/7 -> [T84_6894_11350402720670]
  Demux/8 -> [T84_6895_11351264229999]
  Demux/9 -> [T84_6896_11352362883137]
  Demux/10 -> [T83_6850_11084610973670]
  Demux/11 -> [T83_6851_11085380318587]
  Demux/12 -> [T83_6852_11086383452659]
  Demux/13 -> [T83_6851_11083106068569]
  Demux/14 -> [T83_6852_11083873578369]
  Demux/15 -> [T83_6853_11084874877326]
  Demux/16 -> [T85_7302_11561671089655]
  Demux/17 -> [T85_7303_11565702456143]
  Demux/18 -> [T85_7304_11569968176513]
  Demux/19 -> [T85_7290_11482635956345]
  Demux/20 -> [T85_7291_11486699929756]
  Demux/21 -> [T85_7292_11490998257050]

== system IEEE_39_bus_steady_state/powergui/EquivalentModel19/Sources ==
  Mux : Mux  Inputs=[1 1 1 1 1 1]
  u : Outport  VectorParamsAs1DForOutWhenUnconnected=off
  wires:
  Mux/1 -> u/1
  [T80_6491_9323786358380] -> Mux/1
  [T80_6492_9325151593899] -> Mux/2
  [T80_6493_9326753025418] -> Mux/3
  [T81_6537_9547360139716] -> Mux/4
  [T81_6538_9548818185966] -> Mux/5
  [T81_6539_9550515793944] -> Mux/6

== system IEEE_39_bus_steady_state/powergui/EquivalentModel19/Yout ==
  v,i : Inport
  Demux : Demux  Outputs=[1 1 1 1 1 1 1 1 1]
  tag scope: T60_4974_5505685981297=global, T60_4975_5507935304565=global, T60_4976_5510761424192=global, T83_6849_11086639735874=global, T83_6850_11087410878278=global, T83_6851_11088415809838=global, T84_6895_11349447459880=global, T84_6896_11350306595881=global, T84_6897_11351402875691=global
  wires:
  v,i/1 -> Demux/1
  Demux/1 -> [T60_4974_5505685981297]
  Demux/2 -> [T60_4976_5510761424192]
  Demux/3 -> [T60_4975_5507935304565]
  Demux/4 -> [T83_6849_11086639735874]
  Demux/5 -> [T83_6850_11087410878278]
  Demux/6 -> [T83_6851_11088415809838]
  Demux/7 -> [T84_6895_11349447459880]
  Demux/8 -> [T84_6896_11350306595881]
  Demux/9 -> [T84_6897_11351402875691]

== system IEEE_39_bus_steady_state/powergui/EquivalentModel2/Sources ==
  Mux : Mux  Inputs=[1 1 1 1 1 1]
  u : Outport  VectorParamsAs1DForOutWhenUnconnected=off
  wires:
  Mux/1 -> u/1
  [T78_6382_8917464011002] -> Mux/1
  [T78_6383_8918672859134] -> Mux/2
  [T78_6384_8920111172907] -> Mux/3
  [T79_6439_9115818957624] -> Mux/4
  [T79_6440_9117101452821] -> Mux/5
  [T79_6441_9118616778650] -> Mux/6

== system IEEE_39_bus_steady_state/powergui/EquivalentModel2/Yout ==
  v,i : Inport
  Demux : Demux  Outputs=[1 1 1 1 1 1 1 1 1]
  tag scope: T59_4918_5388541687043=global, T59_4919_5390660345605=global, T59_4920_5393352682653=global, T81_6740_10607628653528=global, T81_6741_10608251627623=global, T81_6742_10609101683448=global, T82_6797_10841378264908=global, T82_6798_10842070998567=global, T82_6799_10842994167347=global
  wires:
  v,i/1 -> Demux/1
  Demux/1 -> [T59_4918_5388541687043]
  Demux/2 -> [T59_4920_5393352682653]
  Demux/3 -> [T59_4919_5390660345605]
  Demux/4 -> [T81_6740_10607628653528]
  Demux/5 -> [T81_6741_10608251627623]
  Demux/6 -> [T81_6742_10609101683448]
  Demux/7 -> [T82_6797_10841378264908]
  Demux/8 -> [T82_6798_10842070998567]
  Demux/9 -> [T82_6799_10842994167347]

== system IEEE_39_bus_steady_state/powergui/EquivalentModel20/Sources ==
  Mux : Mux  Inputs=[1 1 1 1 1 1]
  u : Outport  VectorParamsAs1DForOutWhenUnconnected=off
  wires:
  Mux/1 -> u/1
  [T80_6493_9321698815378] -> Mux/1
  [T80_6494_9323059630758] -> Mux/2
  [T80_6495_9324656642138] -> Mux/3
  [T80_6495_9317813803568] -> Mux/4
  [T80_6496_9319171678340] -> Mux/5
  [T80_6497_9320765749112] -> Mux/6

== system IEEE_39_bus_steady_state/powergui/EquivalentModel20/Yout ==
  v,i : Inport
  Demux : Demux  Outputs=[1 1 1 1 1 1 1 1 1]
  tag scope: T60_4975_5505084877455=global, T60_4976_5507332263379=global, T60_4977_5510156328881=global, T83_6851_11083583583391=global, T83_6852_11084350566391=global, T83_6853_11079145631267=global, T83_6853_11085351338548=global, T83_6854_11079909847120=global, T83_6855_11080907852130=global
  wires:
  v,i/1 -> Demux/1
  Demux/1 -> [T60_4975_5505084877455]
  Demux/2 -> [T60_4977_5510156328881]
  Demux/3 -> [T60_4976_5507332263379]
  Demux/4 -> [T83_6851_11083583583391]
  Demux/5 -> [T83_6852_11084350566391]
  Demux/6 -> [T83_6853_11085351338548]
  Demux/7 -> [T83_6853_11079145631267]
  Demux/8 -> [T83_6854_11079909847120]
  Demux/9 -> [T83_6855_11080907852130]

== system IEEE_39_bus_steady_state/powergui/EquivalentModel21/Sources ==
  Mux : Mux  Inputs=[1 1 1 1 1 1 1 1 1]
  u : Outport  VectorParamsAs1DForOutWhenUnconnected=off
  wires:
  Mux/1 -> u/1
  [T81_6542_9533522927679] -> Mux/1
  [T81_6543_9534973391861] -> Mux/2
  [T81_6544_9536663417772] -> Mux/3
  [T80_6494_9320613660176] -> Mux/4
  [T80_6495_9321972525403] -> Mux/5
  [T80_6496_9323567586631] -> Mux/6
  [T80_6496_9317358720884] -> Mux/7
  [T80_6497_9318714085682] -> Mux/8
  [T80_6498_9320305646479] -> Mux/9

== system IEEE_39_bus_steady_state/powergui/EquivalentModel21/Yout ==
  v,i : Inport
  Demux : Demux  Outputs=[1 1 1 1 1 1 1 1 1 1 1 1]
  tag scope: T60_4976_5504577406946=global, T60_4977_5506822855525=global, T60_4978_5509644866904=global, T83_6852_11082077158031=global, T83_6853_11082842305915=global, T83_6854_11078113991937=global, T83_6854_11083841242956=global, T83_6855_11078875845874=global, T83_6856_11079871488969=global, T84_6900_11334312586380=global, T84_6901_11335164582358=global, T84_6902_11336253722146=global
  wires:
  v,i/1 -> Demux/1
  Demux/1 -> [T60_4976_5504577406946]
  Demux/2 -> [T60_4978_5509644866904]
  Demux/3 -> [T60_4977_5506822855525]
  Demux/4 -> [T84_6900_11334312586380]
  Demux/5 -> [T84_6901_11335164582358]
  Demux/6 -> [T84_6902_11336253722146]
  Demux/7 -> [T83_6852_11082077158031]
  Demux/8 -> [T83_6853_11082842305915]
  Demux/9 -> [T83_6854_11083841242956]
  Demux/10 -> [T83_6854_11078113991937]
  Demux/11 -> [T83_6855_11078875845874]
  Demux/12 -> [T83_6856_11079871488969]

== system IEEE_39_bus_steady_state/powergui/EquivalentModel22/Sources ==
  Mux : Mux  Inputs=[1 1 1 1 1 1 1 1 1]
  u : Outport  VectorParamsAs1DForOutWhenUnconnected=off
  wires:
  Mux/1 -> u/1
  [T78_6384_8913616887885] -> Mux/1
  [T78_6385_8914822069204] -> Mux/2
  [T78_6386_8916256716164] -> Mux/3
  [T79_6438_9116533209114] -> Mux/4
  [T79_6439_9117817960964] -> Mux/5
  [T79_6440_9119335543447] -> Mux/6
  [T78_6385_8910520416563] -> Mux/7
  [T78_6386_8911724419714] -> Mux/8
  [T78_6387_8913157888505] -> Mux/9

== system IEEE_39_bus_steady_state/powergui/EquivalentModel22/Yout ==
  v,i : Inport
  Demux : Demux  Outputs=[1 1 1 1 1 1 1 1 1 1 1 1 1 1 1]
  tag scope: T58_4842_5270914439446=global, T58_4843_5273273122371=global, T58_4844_5275776153227=global, T59_4920_5386183200123=global, T59_4921_5388298027265=global, T59_4922_5390986297206=global, T81_6742_10603063079528=global, T81_6743_10599805563688=global, T81_6743_10603682608327=global, T81_6744_10600423985494=global, T81_6744_10604529218855=global, T81_6745_10601269489028=global, T82_6796_10842598264560=global, T82_6797_10843293120170=global, T82_6798_10844218410902=global
  wires:
  v,i/1 -> Demux/1
  Demux/1 -> [T59_4920_5386183200123]
  Demux/2 -> [T59_4922_5390986297206]
  Demux/3 -> [T59_4921_5388298027265]
  Demux/4 -> [T81_6742_10603063079528]
  Demux/5 -> [T81_6743_10603682608327]
  Demux/6 -> [T81_6744_10604529218855]
  Demux/7 -> [T82_6796_10842598264560]
  Demux/8 -> [T82_6797_10843293120170]
  Demux/9 -> [T82_6798_10844218410902]
  Demux/10 -> [T81_6743_10599805563688]
  Demux/11 -> [T81_6744_10600423985494]
  Demux/12 -> [T81_6745_10601269489028]
  Demux/13 -> [T58_4842_5270914439446]
  Demux/14 -> [T58_4843_5273273122371]
  Demux/15 -> [T58_4844_5275776153227]

== system IEEE_39_bus_steady_state/powergui/EquivalentModel23/Sources ==
  Mux : Mux  Inputs=[2 1 1 1 1 1 1 1 1 1 1 1 1]
  u : Outport  VectorParamsAs1DForOutWhenUnconnected=off
  wires:
  Mux/1 -> u/1
  [T69_5980_8396246211935] -> Mux/1
  [T78_6388_8906438041292] -> Mux/2
  [T78_6389_8907635888984] -> Mux/3
  [T78_6390_8909063202318] -> Mux/4
  [T78_6391_8901000755318] -> Mux/5
  [T78_6392_8902193594219] -> Mux/6
  [T78_6393_8903615898761] -> Mux/7
  [T79_6434_9121682065628] -> Mux/8
  [T79_6435_9122975156203] -> Mux/9
  [T79_6436_9124501077410] -> Mux/10
  [T78_6391_8900534432547] -> Mux/11
  [T78_6392_8901727435258] -> Mux/12
  [T78_6393_8903149903610] -> Mux/13

== system IEEE_39_bus_steady_state/powergui/EquivalentModel23/Yout ==
  v,i : Inport
  Demux : Demux  Outputs=[2 1 1 1 1 1 1 1 1 1 1 1 1 1 1 1 1 1 1 1 1 1 1 1 1]
  tag scope: T59_4891_5389752762087=global, T59_4892_5392257961619=global, T59_4893_5394910822168=global, T59_4922_5384187138966=global, T59_4923_5383325018048=global, T59_4923_5386298134687=global, T59_4924_5385434098060=global, T59_4924_5388982337522=global, T59_4925_5388116267341=global, T60_4969_5510102373887=global, T60_4970_5512361431398=global, T60_4971_5515197872031=global, T69_5975_8327386387613=global, T81_6746_10594428486194=global, T81_6747_10595041124401=global, T81_6748_10595880844336=global, T81_6749_10587607020133=global, T81_6749_10588017342750=global, T81_6750_10588215106049=global, T81_6750_10588625274753=global, T81_6751_10589050273694=global, T81_6751_10589460288485=global, T82_6792_10849523521927=global, T82_6793_10850226218512=global, T82_6794_10851159350220=global
  wires:
  v,i/1 -> Demux/1
  Demux/1 -> [T69_5975_8327386387613]
  Demux/2 -> [T60_4969_5510102373887]
  Demux/3 -> [T60_4971_5515197872031]
  Demux/4 -> [T60_4970_5512361431398]
  Demux/5 -> [T59_4922_5384187138966]
  Demux/6 -> [T59_4924_5388982337522]
  Demux/7 -> [T59_4923_5386298134687]
  Demux/8 -> [T59_4923_5383325018048]
  Demux/9 -> [T59_4925_5388116267341]
  Demux/10 -> [T59_4924_5385434098060]
  Demux/11 -> [T81_6746_10594428486194]
  Demux/12 -> [T81_6747_10595041124401]
  Demux/13 -> [T81_6748_10595880844336]
  Demux/14 -> [T81_6749_10588017342750]
  Demux/15 -> [T81_6750_10588625274753]
  Demux/16 -> [T81_6751_10589460288485]
  Demux/17 -> [T82_6792_10849523521927]
  Demux/18 -> [T82_6793_10850226218512]
  Demux/19 -> [T82_6794_10851159350220]
  Demux/20 -> [T81_6749_10587607020133]
  Demux/21 -> [T81_6750_10588215106049]
  Demux/22 -> [T81_6751_10589050273694]
  Demux/23 -> [T59_4891_5389752762087]
  Demux/24 -> [T59_4892_5392257961619]
  Demux/25 -> [T59_4893_5394910822168]

== system IEEE_39_bus_steady_state/powergui/EquivalentModel24/Sources ==
  Mux : Mux  Inputs=[2 1 1 1 1 1 1]
  u : Outport  VectorParamsAs1DForOutWhenUnconnected=off
  wires:
  Mux/1 -> u/1
  [T69_5978_8400502249876] -> Mux/1
  [T79_6440_9115303093327] -> Mux/2
  [T79_6441_9116583089085] -> Mux/3
  [T79_6442_9118095915475] -> Mux/4
  [T79_6447_9101210114469] -> Mux/5
  [T79_6448_9102478764706] -> Mux/6
  [T79_6449_9103980245576] -> Mux/7

== system IEEE_39_bus_steady_state/powergui/EquivalentModel24/Yout ==
  v,i : Inport
  Demux : Demux  Outputs=[2 1 1 1 1 1 1 1 1 1 1 1 1 1 1 1]
  tag scope: T59_4893_5387849302309=global, T59_4894_5390350362858=global, T59_4895_5392999084424=global, T60_4971_5508051092822=global, T60_4972_5510306228124=global, T60_4973_5513138510124=global, T60_4977_5503408491853=global, T60_4978_5505652050607=global, T60_4979_5508472058246=global, T69_5973_8331621607327=global, T82_6798_10840292117340=global, T82_6799_10840982500754=global, T82_6800_10841903319291=global, T82_6805_10824046655008=global, T82_6806_10824726370129=global, T82_6807_10825636520373=global
  wires:
  v,i/1 -> Demux/1
  Demux/1 -> [T69_5973_8331621607327]
  Demux/2 -> [T60_4971_5508051092822]
  Demux/3 -> [T60_4973_5513138510124]
  Demux/4 -> [T60_4972_5510306228124]
  Demux/5 -> [T60_4977_5503408491853]
  Demux/6 -> [T60_4979_5508472058246]
  Demux/7 -> [T60_4978_5505652050607]
  Demux/8 -> [T82_6798_10840292117340]
  Demux/9 -> [T82_6799_10840982500754]
  Demux/10 -> [T82_6800_10841903319291]
  Demux/11 -> [T82_6805_10824046655008]
  Demux/12 -> [T82_6806_10824726370129]
  Demux/13 -> [T82_6807_10825636520373]
  Demux/14 -> [T59_4893_5387849302309]
  Demux/15 -> [T59_4894_5390350362858]
  Demux/16 -> [T59_4895_5392999084424]

== system IEEE_39_bus_steady_state/powergui/EquivalentModel25/Sources ==
  Mux : Mux  Inputs=[1 1 1 1 1 1 1 1 1]
  u : Outport  VectorParamsAs1DForOutWhenUnconnected=off
  wires:
  Mux/1 -> u/1
  [T78_6386_8909941564649] -> Mux/1
  [T78_6387_8911143079154] -> Mux/2
  [T78_6388_8912574059301] -> Mux/3
  [T79_6435_9120132345368] -> Mux/4
  [T79_6436_9121423098361] -> Mux/5
  [T79_6437_9122946681986] -> Mux/6
  [T78_6387_8907019955345] -> Mux/7
  [T78_6388_8908220291682] -> Mux/8
  [T78_6389_8909650093660] -> Mux/9

== system IEEE_39_bus_steady_state/powergui/EquivalentModel25/Yout ==
  v,i : Inport
  Demux : Demux  Outputs=[1 1 1 1 1 1 1 1 1 1 1 1 1 1 1]
  tag scope: T58_4843_5269941752269=global, T58_4844_5272298411606=global, T58_4845_5274799418875=global, T59_4921_5385139866324=global, T59_4922_5387252777756=global, T59_4923_5389939014144=global, T81_6744_10598663023750=global, T81_6745_10595573864281=global, T81_6745_10599279107253=global, T81_6746_10596188840790=global, T81_6746_10600122272485=global, T81_6747_10597030899028=global, T82_6793_10847479681989=global, T82_6794_10848180180525=global, T82_6795_10849111114184=global
  wires:
  v,i/1 -> Demux/1
  Demux/1 -> [T59_4921_5385139866324]
  Demux/2 -> [T59_4923_5389939014144]
  Demux/3 -> [T59_4922_5387252777756]
  Demux/4 -> [T81_6744_10598663023750]
  Demux/5 -> [T81_6745_10599279107253]
  Demux/6 -> [T81_6746_10600122272485]
  Demux/7 -> [T82_6793_10847479681989]
  Demux/8 -> [T82_6794_10848180180525]
  Demux/9 -> [T82_6795_10849111114184]
  Demux/10 -> [T81_6745_10595573864281]
  Demux/11 -> [T81_6746_10596188840790]
  Demux/12 -> [T81_6747_10597030899028]
  Demux/13 -> [T58_4843_5269941752269]
  Demux/14 -> [T58_4844_5272298411606]
  Demux/15 -> [T58_4845_5274799418875]

== system IEEE_39_bus_steady_state/powergui/EquivalentModel26/Sources ==
  Mux : Mux  Inputs=[1 1 1 1 1 1 1 1 1]
  u : Outport  VectorParamsAs1DForOutWhenUnconnected=off
  wires:
  Mux/1 -> u/1
  [T78_6392_8900412580193] -> Mux/1
  [T78_6393_8901602930450] -> Mux/2
  [T78_6394_8903022746347] -> Mux/3
  [T78_6392_8899946394219] -> Mux/4
  [T78_6393_8901136908285] -> Mux/5
  [T78_6394_8902556887992] -> Mux/6
  [T78_6396_8894141946667] -> Mux/7
  [T78_6397_8895325127106] -> Mux/8
  [T78_6398_8896737773187] -> Mux/9

== system IEEE_39_bus_steady_state/powergui/EquivalentModel26/Yout ==
  v,i : Inport
  Demux : Demux  Outputs=[1 1 1 1 1 1 1 1 1 1 1 1 1 1 1]
  tag scope: T59_4924_5382553503571=global, T59_4925_5381872595535=global, T59_4925_5384660667873=global, T59_4926_5383977844126=global, T59_4926_5387340803600=global, T59_4927_5386655946300=global, T81_6750_10586455965750=global, T81_6750_10586866161577=global, T81_6751_10587061713364=global, T81_6751_10587471755278=global, T81_6752_10587894542707=global, T81_6752_10588304430707=global, T81_6754_10579145518194=global, T81_6755_10579744375216=global, T81_6756_10580570313966=global
  wires:
  v,i/1 -> Demux/1
  Demux/1 -> [T59_4924_5382553503571]
  Demux/2 -> [T59_4926_5387340803600]
  Demux/3 -> [T59_4925_5384660667873]
  Demux/4 -> [T59_4925_5381872595535]
  Demux/5 -> [T59_4927_5386655946300]
  Demux/6 -> [T59_4926_5383977844126]
  Demux/7 -> [T81_6750_10586866161577]
  Demux/8 -> [T81_6751_10587471755278]
  Demux/9 -> [T81_6752_10588304430707]
  Demux/10 -> [T81_6750_10586455965750]
  Demux/11 -> [T81_6751_10587061713364]
  Demux/12 -> [T81_6752_10587894542707]
  Demux/13 -> [T81_6754_10579145518194]
  Demux/14 -> [T81_6755_10579744375216]
  Demux/15 -> [T81_6756_10580570313966]

== system IEEE_39_bus_steady_state/powergui/EquivalentModel3/Sources ==
  Mux : Mux  Inputs=[2 1 1 1 1 1 1]
  u : Outport  VectorParamsAs1DForOutWhenUnconnected=off
  wires:
  Mux/1 -> u/1
  [T69_5988_8380948991458] -> Mux/1
  [T80_6482_9339833862152] -> Mux/2
  [T80_6483_9341215129519] -> Mux/3
  [T80_6484_9342832592886] -> Mux/4
  [T80_6483_9336522133340] -> Mux/5
  [T80_6484_9337902210315] -> Mux/6
  [T80_6485_9339518483290] -> Mux/7

== system IEEE_39_bus_steady_state/powergui/EquivalentModel3/Yout ==
  v,i : Inport
  Demux : Demux  Outputs=[2 1 1 1 1 1 1 1 1 1 1 1 1 1 1 1]
  tag scope: T60_4941_5510144590879=global, T60_4942_5512794273627=global, T60_4943_5515594932709=global, T60_4969_5510096000506=global, T60_4970_5512355010497=global, T60_4971_5515191400746=global, T61_5019_5635481711825=global, T61_5020_5637883269475=global, T61_5021_5640865767792=global, T69_5983_8312172440043=global, T83_6840_11105892199354=global, T83_6841_11102419961205=global, T83_6841_11106678427917=global, T83_6842_11103205069594=global, T83_6842_11107698445636=global, T83_6843_11104223967141=global
  wires:
  v,i/1 -> Demux/1
  Demux/1 -> [T69_5983_8312172440043]
  Demux/2 -> [T60_4969_5510096000506]
  Demux/3 -> [T60_4971_5515191400746]
  Demux/4 -> [T60_4970_5512355010497]
  Demux/5 -> [T61_5019_5635481711825]
  Demux/6 -> [T61_5021_5640865767792]
  Demux/7 -> [T61_5020_5637883269475]
  Demux/8 -> [T83_6840_11105892199354]
  Demux/9 -> [T83_6841_11106678427917]
  Demux/10 -> [T83_6842_11107698445636]
  Demux/11 -> [T83_6841_11102419961205]
  Demux/12 -> [T83_6842_11103205069594]
  Demux/13 -> [T83_6843_11104223967141]
  Demux/14 -> [T60_4941_5510144590879]
  Demux/15 -> [T60_4942_5512794273627]
  Demux/16 -> [T60_4943_5515594932709]

== system IEEE_39_bus_steady_state/powergui/EquivalentModel4/Sources ==
  Mux : Mux  Inputs=[2 1 1 1]
  u : Outport  VectorParamsAs1DForOutWhenUnconnected=off
  wires:
  Mux/1 -> u/1
  [T69_5994_8371289353951] -> Mux/1
  [T81_6541_9535203805086] -> Mux/2
  [T81_6542_9536656275750] -> Mux/3
  [T81_6543_9538348308142] -> Mux/4

== system IEEE_39_bus_steady_state/powergui/EquivalentModel4/Yout ==
  v,i : Inport
  Demux : Demux  Outputs=[2 1 1 1 1 1 1 1 1 1 1 1 1]
  tag scope: T59_4898_5384094177282=global, T59_4899_5386585065885=global, T59_4900_5389223615506=global, T60_4970_5509034939760=global, T60_4971_5511292107446=global, T60_4972_5514126544339=global, T60_4976_5503917510441=global, T60_4977_5506163006540=global, T60_4978_5508985068302=global, T69_5989_8302575257217=global, T84_6899_11336408406345=global, T84_6900_11337262291824=global, T84_6901_11338353321113=global
  wires:
  v,i/1 -> Demux/1
  Demux/1 -> [T69_5989_8302575257217]
  Demux/2 -> [T60_4976_5503917510441]
  Demux/3 -> [T60_4978_5508985068302]
  Demux/4 -> [T60_4977_5506163006540]
  Demux/5 -> [T60_4970_5509034939760]
  Demux/6 -> [T60_4972_5514126544339]
  Demux/7 -> [T60_4971_5511292107446]
  Demux/8 -> [T84_6899_11336408406345]
  Demux/9 -> [T84_6900_11337262291824]
  Demux/10 -> [T84_6901_11338353321113]
  Demux/11 -> [T59_4898_5384094177282]
  Demux/12 -> [T59_4899_5386585065885]
  Demux/13 -> [T59_4900_5389223615506]
